simulink model "euler321_I2B_12B"  (R2021a)
settings: Solver=ode3  StartTime=0.0  StopTime=10.0  FixedStep=0.01  RelTol=1e-3  EnableMultiTasking=on
model workspace (MAT data in the model file):
  X = [2.82349418676 1.62907668459 2.19953938585 0.797466441882 0.483707410954 -2.31662366019 2.91825739244 3.13458055029 0.41915422695 -3.04934593888 -1.84933917806 2.61583239987 ... (7007 elements, 1x7007)]
  cs : handle (value not decoded)
  curPath = '/Users/khouloud.gaaloul/Documents/Projects/QRA-LocalSearch/Local Search Algorithms/Problems'
  d = 4004
  hws = []
  i = 6
  model_cs : handle (value not decoded)
  modelpath = '/Users/khouloud.gaaloul/Documents/Projects/QRA-LocalSearch/Simulink Models/9_euler/'
  req = 'R1'
  t = [0 0.01 0.02 0.03 0.04 0.05 0.06 0.07 0.08 0.09 0.1 0.11 ... (1001 elements, 1x1001)]
  var.time = [0 0.01 0.02 0.03 0.04 0.05 0.06 0.07 0.08 0.09 0.1 0.11 ... (1001 elements, 1001x1)]
  var.signals(1).values = [2.82349418676 1.62907668459 2.19953938585 0.797466441882 0.483707410954 -2.31662366019 2.91825739244 3.13458055029 0.41915422695 -3.04934593888 -1.84933917806 2.61583239987 ... (1001 elements, 1001x1)]
  var.signals(2).values = [3.04998762921 0.973668245912 1.48181435148 1.27106577271 0.771739655209 0.909425533572 -0.854881070359 2.76966099427 -1.77565085343 -1.11950162472 0.871268475432 -1.97360358899 ... (1001 elements, 1001x1)]
  var.signals(3).values = [-2.40817312386 3.05698045978 0.435242644232 -0.0658968366341 -1.0968175547 -2.24569039289 3.11022732441 -2.84243410587 1.40475817305 -1.27211547445 -0.852306425564 2.65873983624 ... (1001 elements, 1001x1)]
  var.signals(4).values = [70.4153624458 71.7517202331 63.2784478543 65.4542388444 3.67143822843 41.2400805015 29.147835644 39.898535832 38.0558015955 24.7120341708 69.7836438558 8.94889286659 ... (3003 elements, 1001x3)]
  var.signals(5).values = [1.24546093453 -0.587654372768 0.780959752949 2.00351624985 -1.61511386441 -0.819932043746 2.30877567704 2.55059507567 1.04678835055 -2.79515743554 2.77427406088 -0.390972168213 ... (1001 elements, 1001x1)]
libraries: sharedutil x9, sldvlib x9, dspmtrx3 x2
(part 1 of 2)
settings Model: Creator=elliocm  LastModifiedBy=yangy
settings SolverCC: AlgebraicLoopSolver=TrustRegion
settings DataIOCC: ExternalInput=var  LimitDataPoints=on  LoadExternalInput=on  SaveFormat=StructureWithTime  SignalLoggingSaveFormat=ModelDataLogs  ReturnWorkspaceOutputs=off
settings OptimizationCC: DefaultParameterBehavior=Inlined  EnhancedBackFolding=on  PassReuseOutputArgsAs=Individual arguments  ExpressionDepthLimit=2147483647  ZeroExternalMemoryAtStartup=off  ZeroInternalMemoryAtStartup=off  OptimizeBlockOrder=speed  DifferentSizesBufferReuse=on  OptimizationCustomize=off  EfficientTunableParamExpr=on
settings DebuggingCC: UnderspecifiedInitializationDetection=Classic  MergeDetectMultiDrivingBlocksExec=none  SolverPrmCheckMsg=warning  ParameterTunabilityLossMsg=error  FcnCallInpInsideContextMsg=warning  StateNameClashWarn=warning  SFUnexpectedBacktrackingDiag=warning  SFNoUnconditionalDefaultTransitionDiag=warning  SFExecutionAtInitializationDiag=none  SFMachineParentedDataDiag=warning  ArithmeticOperatorsInVariantConditions=warning
settings HardwareCC: ProdBitPerPointer=32  ProdBitPerSizeT=32  ProdBitPerPtrDiffT=32  ProdLargestAtomicFloat=None  ProdIntDivRoundTo=Undefined  ProdEndianess=Unspecified  ProdWordSize=32  ProdHWDeviceType=32-bit Generic
settings ModelReferenceCC: PropagateSignalLabelsOutOfModel=off
settings SFSimCC: SimUseLocalCustomCode=off  MATLABDynamicMemAlloc=off  CustomCodeUndefinedFunction=UseInterfaceOnly
settings RTWCC: SystemTargetFile=ert.tlc  GenCodeOnly=on  TemplateMakefile=ert_default_tmf  RTWUseLocalCustomCode=off
settings CodeAppCC: GenerateComments=off  IgnoreCustomStorageClasses=off  OperatorAnnotations=on  SimulinkDataObjDesc=on  SFDataObjDesc=on  SimulinkBlockComments=off
settings ERTTargetCC: GenerateSampleERTMain=on  InlinedParameterPlacement=NonHierarchical  ERTCustomFileTemplate=example_file_process.tlc
settings ConfigComp: CovMetricSettings=dw  CovSaveCumulativeToWorkspaceVar=on  CovSaveSingleToWorkspaceVar=on  CovExternalEMLEnable=off

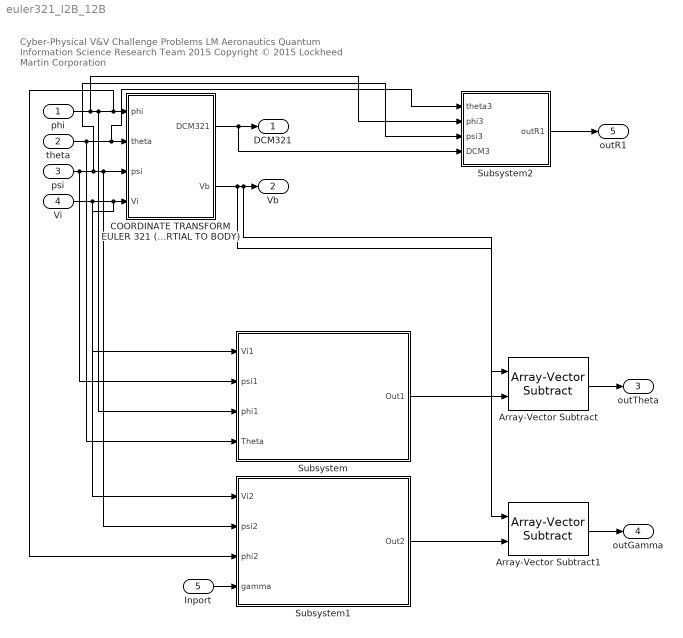
== system euler321_I2B_12B ==
  note: Cyber-Physical V&V Challenge Problems
      | LM Aeronautics Quantum Information Science Research Team 2015
      | Copyright © 2015 Lockheed Martin Corporation
  phi : Inport  OutDataTypeStr=double
  theta : Inport  Port=2  OutDataTypeStr=double
  psi : Inport  Port=3  OutDataTypeStr=double
  Vi : Inport  Port=4  OutDataTypeStr=double  PortDimensions=3
  Inport : Inport  Port=5
  Array-Vector Subtract : dspmtrx3/Array-Vector Subtract  Dimension=1  V_Source=Input port  V_VectFromMask=[0.5 0.25]  prodOutputSignedness=Auto  roundingMode=Floor  overflowMode=off  firstCoeffSignedness=Auto  firstCoeffDataTypeStr=Inherit: Same word length as input  firstCoeffMin=[]  firstCoeffMax=[]  firstCoeffLastDataTypeStr=Inherit: Same word length as input  accumSignedness=Auto  outputSignedness=Auto  outputDataTypeStr=Inherit: Same as accumulator  outputMin=[]  outputMax=[]  outputLastDataTypeStr=Inherit: Same as accumulator
      settings: SourceProductBaseCode=DS
  Array-Vector Subtract1 : dspmtrx3/Array-Vector Subtract  Dimension=1  V_Source=Input port  V_VectFromMask=[0.5 0.25]  prodOutputSignedness=Auto  roundingMode=Floor  overflowMode=off  firstCoeffSignedness=Auto  firstCoeffDataTypeStr=Inherit: Same word length as input  firstCoeffMin=[]  firstCoeffMax=[]  firstCoeffLastDataTypeStr=Inherit: Same word length as input  accumSignedness=Auto  outputSignedness=Auto  outputDataTypeStr=Inherit: Same as accumulator  outputMin=[]  outputMax=[]  outputLastDataTypeStr=Inherit: Same as accumulator
      settings: SourceProductBaseCode=DS
  COORDINATE TRANSFORM EULER 321 (INERTIAL TO BODY) : Subsystem
  Subsystem : Subsystem
  Subsystem1 : Subsystem
  Subsystem2 : Subsystem
  DCM321 : Outport  VectorParamsAs1DForOutWhenUnconnected=off
  Vb : Outport  Port=2  VectorParamsAs1DForOutWhenUnconnected=off
  outTheta : Outport  Port=3  VectorParamsAs1DForOutWhenUnconnected=off
  outGamma : Outport  Port=4  VectorParamsAs1DForOutWhenUnconnected=off
  outR1 : Outport  Port=5  VectorParamsAs1DForOutWhenUnconnected=off
  wires:
  Vi/1 -> Subsystem/1(Vi1), Subsystem1/1(Vi2), COORDINATE TRANSFORM EULER 321 (INERTIAL TO BODY)/4(Vi)
  Subsystem/1(Out1) -> Array-Vector Subtract/2
  Array-Vector Subtract/1 -> outTheta/1
  Array-Vector Subtract1/1 -> outGamma/1
  COORDINATE TRANSFORM EULER 321 (INERTIAL TO BODY)/2(Vb) -> Array-Vector Subtract1/1, Array-Vector Subtract/1, Vb/1
  Subsystem1/1(Out2) -> Array-Vector Subtract1/2
  Inport/1 -> Subsystem1/4(gamma)
  COORDINATE TRANSFORM EULER 321 (INERTIAL TO BODY)/1(DCM321) -> Subsystem2/4(DCM3), DCM321/1
  phi/1 -> Subsystem2/2(phi3), Subsystem/3(phi1), Subsystem1/3(phi2), COORDINATE TRANSFORM EULER 321 (INERTIAL TO BODY)/1(phi)
  psi/1 -> Subsystem/2(psi1), Subsystem2/3(psi3), Subsystem1/2(psi2), COORDINATE TRANSFORM EULER 321 (INERTIAL TO BODY)/3(psi)
  theta/1 -> Subsystem/4(Theta), Subsystem2/1(theta3), COORDINATE TRANSFORM EULER 321 (INERTIAL TO BODY)/2(theta)
  Subsystem2/1(outR1) -> outR1/1
